simulink model "SingleSOC_Batery_Model"  (R2016b)
settings: Solver=VariableStepAuto  StartTime=0  StopTime=time_buffer(indexes(1).end)  RelTol=1e-3
values from neighbouring files (symbols this model uses):
  R0 = Average_R0(meas.Current,meas.Voltage)    [Copy_of_generate_dynamic_parameters_relaxation.m]    (also in Optimization.m = vOpt(5).Value; Semi-Automatic Li Ion battery  RC model parameters estimator.m = vOpt(5).Value; generate_dynamic_parameters_relaxation.m = Average_R0(meas.Current, meas.Voltage))
  R1 = R1_table(indice)    [Copy_of_generate_dynamic_parameters_relaxation.m]    (also in Optimization.m = vOpt(1).Value; Semi-Automatic Li Ion battery  RC model parameters estimator.m = vOpt(1).Value; generate_dynamic_parameters_relaxation.m)
  R2 = R2_table(indice)    [Copy_of_generate_dynamic_parameters_relaxation.m]    (also in Optimization.m = vOpt(3).Value; Semi-Automatic Li Ion battery  RC model parameters estimator.m = vOpt(3).Value; generate_dynamic_parameters_relaxation.m)
libraries: fl_lib x9, nesl_utility x4
settings Model: Creator=Fededc88  LastModifiedBy=Fededc88

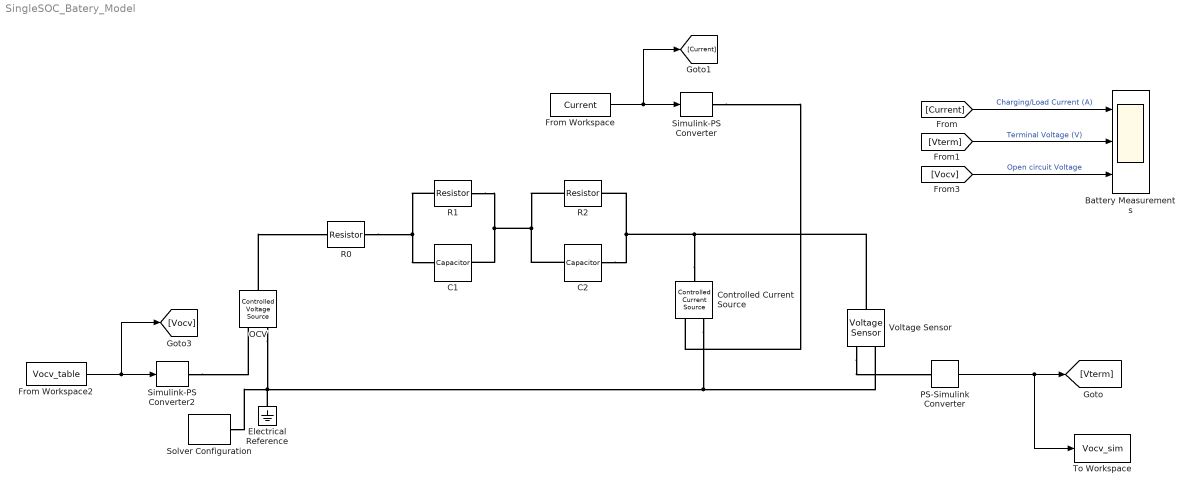
== system SingleSOC_Batery_Model ==
  Battery Measurements : Scope  NumInputPorts=3
  C1 : fl_lib/Electrical/Electrical Elements/Capacitor  c=C1 F  r=0 Ohm  g=0 1/Ohm  i_specify=off  i_priority=None  i=0 A  v_specify=off  v_priority=None  v=0 V  vc_specify=off  vc_priority=High  vc=0 V
  C2 : fl_lib/Electrical/Electrical Elements/Capacitor  c=C2 F  r=0 Ohm  g=0 1/Ohm  i_specify=off  i_priority=None  i=0 A  v_specify=off  v_priority=None  v=0 V  vc_specify=off  vc_priority=High  vc=0 V
  Controlled Current Source : fl_lib/Electrical/Electrical Sources/Controlled Current Source
  Electrical Reference : fl_lib/Electrical/Electrical Elements/Electrical Reference
  From Workspace : FromWorkspace  VariableName=Current  OutDataTypeStr=double  SampleTime=0
  From Workspace2 : FromWorkspace  VariableName=Vocv_table  SampleTime=0
  OCV : fl_lib/Electrical/Electrical Sources/Controlled Voltage Source
  PS-Simulink Converter : nesl_utility/PS-Simulink Converter  PhysicalDomain=network_engine_domain  SubClassName=ps_output  LeftPortType=input  RightPortType=output  PseudoPeriodic=off  Frequencies=[]  Unit=V  AffineConversion=off
  R0 : fl_lib/Electrical/Electrical Elements/Resistor  R=R0 Ohm  i_specify=off  i_priority=None  i=0 A  v_specify=off  v_priority=None  v=0 V
  R1 : fl_lib/Electrical/Electrical Elements/Resistor  R=R1 Ohm  i_specify=off  i_priority=None  i=0 A  v_specify=off  v_priority=None  v=0 V
  R2 : fl_lib/Electrical/Electrical Elements/Resistor  R=R2 Ohm  i_specify=off  i_priority=None  i=0 A  v_specify=off  v_priority=None  v=0 V
  Simulink-PS Converter : nesl_utility/Simulink-PS Converter  PhysicalDomain=network_engine_domain  SubClassName=ps_input  LeftPortType=input  RightPortType=output  PseudoPeriodic=off  Frequencies=[]  NoiseDistribution=none  NoiseParameters=[]  Unit=A  AffineConversion=off  InputFiltering=off  SimscapeFilterOrder=1  InputFilterTimeConstant=.001  UdotUserProvided=1
  Simulink-PS Converter2 : nesl_utility/Simulink-PS Converter  PhysicalDomain=network_engine_domain  SubClassName=ps_input  LeftPortType=input  RightPortType=output  PseudoPeriodic=off  Frequencies=[]  NoiseDistribution=none  NoiseParameters=[]  Unit=V  AffineConversion=off  InputFiltering=off  SimscapeFilterOrder=1  InputFilterTimeConstant=.001  UdotUserProvided=1
  Solver Configuration : nesl_utility/Solver Configuration  PhysicalDomain=network_engine_domain  SubClassName=solver  LeftPortType=input  RightPortType=generic  Accelerate=off  Tones=[]  Harmonics=[]  SimulateNoise=off  Profile=off  UseLocalSampling=off  EnableSwitchedLinearOptims=on  FrequencyDomain=off  UseCCode=off  RelTol=0.001  AbsTol=1e-06  MinStep=1e-09  ToWorkspace=off  RevertToSquareIcSolve=off  NumHomotopyIterations=100  PhasorMode=off  PhasorModeNumHarmonics=1  OverrideAbsTol=off  DoDC=off  ResidualTolerance=1  UseLocalSolver=on  LocalSolverChoice=NE_BACKWARD_EULER_ADVANCER  LocalSolverSampleTime=0.01  DoFixedCost=on  MaxNonlinIter=3  MaxModeIter=2  LinearAlgebra=Full  DelaysMemoryBudget=1024  AutomaticFiltering=off  FilteringTimeConstant=0.001
  To Workspace : ToWorkspace  VariableName=Vocv_sim  SaveFormat=Timeseries  SampleTime=-1
  Voltage Sensor : fl_lib/Electrical/Electrical Sensors/Voltage Sensor
  wires:
  From Workspace2/1 -> [Vocv], Simulink-PS Converter2/1
  [Current] -> Battery Measurements/1  "Charging/Load Current (A)"
  [Vterm] -> Battery Measurements/2  "Terminal Voltage (V)"
  From Workspace/1 -> [Current], Simulink-PS Converter/1
  PS-Simulink Converter/1 -> To Workspace/1, [Vterm]
  [Vocv] -> Battery Measurements/3  "Open circuit Voltage"
  connections:
  OCV/LConn1 -- R0/LConn1
  Simulink-PS Converter2/RConn1 -- OCV/RConn1
  Solver Configuration/RConn1 -- Voltage Sensor/RConn2 -- Controlled Current Source/RConn2 -- Electrical Reference/LConn1 -- OCV/RConn2
  Voltage Sensor/RConn1 -- PS-Simulink Converter/LConn1
  Simulink-PS Converter/RConn1 -- Controlled Current Source/RConn1
  R1/RConn1 -- R2/LConn1 -- C2/LConn1 -- C1/RConn1
  R0/RConn1 -- C1/LConn1 -- R1/LConn1
  Controlled Current Source/LConn1 -- C2/RConn1 -- R2/RConn1 -- Voltage Sensor/LConn1
